simulink model "gm_parallel_8_prediction_and_cost_function"  (R2022a)
settings: Solver=FixedStepDiscrete  StartTime=0.0  StopTime=10.0  RelTol=1e-3
undefined symbols (not defined in the file or in its folder): f_c, L_d, L_q, L_x, L_y, p, psi_pm, R_ph
libraries: hdlmdlgenlib x42, hdlsllib x5
(part 1 of 7)
settings Model: Creator=Andre Merx  LastModifiedBy=Andre Merx
settings SolverCC: AlgebraicLoopSolver=TrustRegion
settings DataIOCC: LimitDataPoints=on  SaveOutput=off  SaveTime=off
settings OptimizationCC: BlockReduction=off  ConditionallyExecuteInputs=off  DefaultParameterBehavior=Inlined  LifeSpan=inf
settings DebuggingCC: AlgebraicLoopMsg=error  InheritedTsInSrcMsg=none  SingleTaskRateTransMsg=error  UnconnectedInputMsg=warning  UnconnectedOutputMsg=warning  UnconnectedLineMsg=warning  AllowSymbolicDim=off  StrictBusMsg=ErrorOnBusTreatedAsVector  SFUnexpectedBacktrackingDiag=warning  SFNoUnconditionalDefaultTransitionDiag=warning  SFExecutionAtInitializationDiag=none  SFMachineParentedDataDiag=warning  ArithmeticOperatorsInVariantConditions=warning
settings HardwareCC: ProdBitPerPointer=32  ProdBitPerSizeT=32  ProdBitPerPtrDiffT=32  ProdLargestAtomicFloat=None  ProdIntDivRoundTo=Undefined  ProdEndianess=Unspecified  ProdWordSize=32  ProdHWDeviceType=ASIC/FPGA->ASIC/FPGA  ProdEqTarget=off
settings SFSimCC: SimUseLocalCustomCode=off  CustomCodeUndefinedFunction=UseInterfaceOnly
settings RTWCC: RTWUseLocalCustomCode=off
settings CodeAppCC: StateflowObjectComments=on
settings GRTTargetCC: TargetLangStandard=C89/C90 (ANSI)
settings ConfigComp: CovScope=ReferencedModels  CovMetricSettings=dw  CovSaveCumulativeToWorkspaceVar=on  CovSaveSingleToWorkspaceVar=on  CovExternalEMLEnable=off  CovSFcnEnable=off

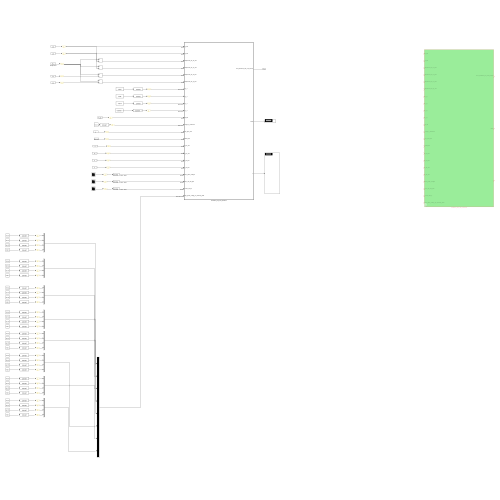
[thumbnail: Simulink's stored preview of the top-level diagram]
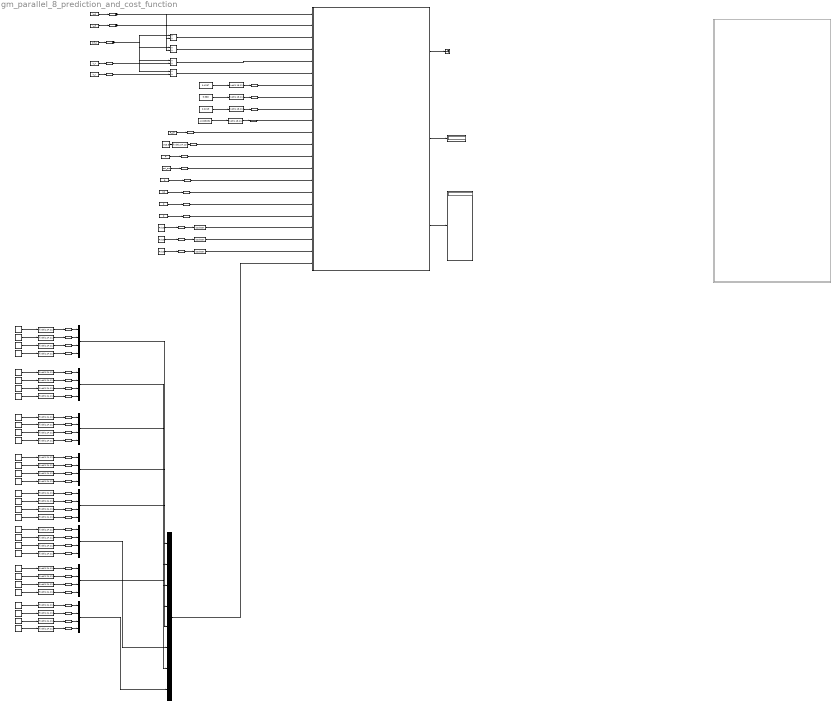
== system gm_parallel_8_prediction_and_cost_function ==
  Constant1 : Constant  Value=L_d  OutDataTypeStr=single  SampleTime=-1
  Constant10 : Constant  Value=0  OutDataTypeStr=single  SampleTime=-1
  Constant{11,30,34,38,42,46,70,74} (8 alike) : Constant  Value=-163.1
  Constant12 : Constant  Value=L_x  OutDataTypeStr=single  SampleTime=-1
  Constant13 : Constant  Value=L_y  OutDataTypeStr=single  SampleTime=-1
  Constant18 : Constant  Value=0.4297
  Constant19 : Constant  Value=R_ph  OutDataTypeStr=single  SampleTime=-1
  Constant2 : Constant  Value=L_q  OutDataTypeStr=single  SampleTime=-1
  Constant20 : Constant  Value=313.3
  Constant21 : Constant  Value=p  OutDataTypeStr=single  SampleTime=-1
  Constant22 : Constant  Value=9.988
  Constant23 : Constant  Value=0.2219
  Constant24 : Constant  Value=psi_pm  OutDataTypeStr=single  SampleTime=-1
  Constant25 : Constant  Value=-0.003051
  Constant{4,31,35,39,43,47,71,75} (8 alike) : Constant  Value=173.9
  Constant{5,32,36,40,44,48,72,76} (8 alike) : Constant  Value=72.19
  Constant{6,33,37,41,45,49,73,77} (8 alike) : Constant  Value=-94.17
  Constant7 : Constant  Value=0  OutDataTypeStr=single  SampleTime=-1
  Constant8 : Constant  Value=10  OutDataTypeStr=single  SampleTime=-1
  Constant9 : Constant  Value=0  OutDataTypeStr=single  SampleTime=-1
  Data Type Conversion{2..6,10,20..21,25..41,62..69} (33 alike) : DataTypeConversion  OutDataTypeStr=fixdt(1,24,11)  SaturateOnIntegerOverflow=off  RndMeth=Floor
  Data Type Conversion{12..15} (4 alike) : DataTypeConversion  OutDataTypeStr=fixdt(1,18,11)  SaturateOnIntegerOverflow=off  RndMeth=Floor
  Data Type Conversion22 : DataTypeConversion  OutDataTypeStr=boolean  SaturateOnIntegerOverflow=off  RndMeth=Floor
  Data Type Conversion23 : DataTypeConversion  OutDataTypeStr=boolean  SaturateOnIntegerOverflow=off  RndMeth=Floor
  Data Type Conversion24 : DataTypeConversion  OutDataTypeStr=boolean  SaturateOnIntegerOverflow=off  RndMeth=Floor
  Display : Display
  Display1 : Display
  Divide{,1..3} (4 alike) : Product  Inputs=*/  RndMeth=Zero  SaturateOnIntegerOverflow=on
  Mux{,1..7} (8 alike) : Mux
  Mux16 : Mux  Inputs=8
  Prediction_and_cost_function1 : Subsystem  TreatAsAtomicUnit=on
  Prediction_and_cost_function2 : Subsystem  Commented=on  TreatAsAtomicUnit=on
  Pulse Generator4 : DiscretePulseGenerator  PulseType=Time based  Period=1/f_c
  Pulse Generator5 : DiscretePulseGenerator  PulseType=Time based  Period=1/f_c
  Pulse Generator6 : DiscretePulseGenerator  PulseType=Time based  Period=1/f_c
  Rate Transition{3..8,12..15,17..28,33..54,75..82} (52 alike) : RateTransition  OutPortSampleTime=Rt
  SampleTime : Constant  Value=1/f_c  OutDataTypeStr=single  SampleTime=-1
  Terminator : Terminator
  wires:
  Mux5/1 -> Mux16/6
  Constant13/1 -> Rate Transition21/1
  SampleTime/1 -> Rate Transition19/1
  Rate Transition20/1 -> Divide2/2
  Constant49/1 -> Data Type Conversion40/1
  Data Type Conversion24/1 -> Prediction_and_cost_function1/19(done_phase_voltages)  "curent_valid_in"
  Constant4/1 -> Data Type Conversion10/1
  Constant18/1 -> Data Type Conversion12/1
  Divide/1 -> Prediction_and_cost_function1/3(SampleTime_div_Ld_AXI)
  Constant10/1 -> Rate Transition15/1
  Constant1/1 -> Rate Transition5/1
  Constant25/1 -> Data Type Conversion15/1
  Constant31/1 -> Data Type Conversion3/1
  Rate Transition33/1 -> Mux1/2
  Data Type Conversion10/1 -> Rate Transition3/1
  Divide3/1 -> Prediction_and_cost_function1/6(SampleTime_div_Ly_AXI)
  Rate Transition28/1 -> Prediction_and_cost_function1/10(iy_k_1)
  Rate Transition26/1 -> Prediction_and_cost_function1/9(ix_k_1)
  Constant6/1 -> Data Type Conversion4/1
  Constant8/1 -> Rate Transition13/1
  Data Type Conversion40/1 -> Rate Transition53/1
  Constant39/1 -> Data Type Conversion30/1
  Rate Transition27/1 -> Prediction_and_cost_function1/14(psiPM_AXI)
  Rate Transition21/1 -> Divide3/2
  Data Type Conversion15/1 -> Rate Transition28/1
  Constant7/1 -> Rate Transition12/1
  Rate Transition37/1 -> Data Type Conversion23/1
  Data Type Conversion22/1 -> Prediction_and_cost_function1/20(done_vsd_and_park)  "curent_valid_in"
  Rate Transition17/1 -> Prediction_and_cost_function1/7(id_k_1)
  Pulse Generator6/1 -> Rate Transition37/1
  Rate Transition36/1 -> Data Type Conversion22/1
  Constant47/1 -> Data Type Conversion38/1
  Rate Transition8/1 -> Mux/4
  Pulse Generator5/1 -> Rate Transition36/1
  Data Type Conversion34/1 -> Rate Transition47/1
  Rate Transition13/1 -> Prediction_and_cost_function1/16(iq_ref_AXI)
  Data Type Conversion14/1 -> Rate Transition26/1
  Constant77/1 -> Data Type Conversion68/1
  Rate Transition19/1 -> Divide/1, Divide2/1, Divide3/1, Divide1/1
  Pulse Generator4/1 -> Rate Transition35/1
  Constant22/1 -> Data Type Conversion13/1
  Data Type Conversion25/1 -> Rate Transition38/1
  Data Type Conversion31/1 -> Rate Transition44/1
  Constant20/1 -> Data Type Conversion5/1
  Data Type Conversion21/1 -> Rate Transition34/1
  Data Type Conversion20/1 -> Rate Transition33/1
  Rate Transition46/1 -> Mux4/4
  Constant35/1 -> Data Type Conversion26/1
  Data Type Conversion35/1 -> Rate Transition48/1
  Constant34/1 -> Data Type Conversion29/1
  Data Type Conversion33/1 -> Rate Transition46/1
  Data Type Conversion32/1 -> Rate Transition45/1
  Constant11/1 -> Data Type Conversion6/1
  Rate Transition3/1 -> Mux/1
  Constant36/1 -> Data Type Conversion27/1
  Data Type Conversion39/1 -> Rate Transition52/1
  Data Type Conversion27/1 -> Rate Transition40/1
  Rate Transition79/1 -> Mux6/1
  Data Type Conversion30/1 -> Rate Transition43/1
  Data Type Conversion37/1 -> Rate Transition50/1
  Data Type Conversion41/1 -> Rate Transition54/1
  Constant48/1 -> Data Type Conversion39/1
  Constant45/1 -> Data Type Conversion36/1
  Constant44/1 -> Data Type Conversion35/1
  Constant43/1 -> Data Type Conversion34/1
  Constant32/1 -> Data Type Conversion20/1
  Data Type Conversion12/1 -> Rate Transition17/1
  Rate Transition35/1 -> Data Type Conversion24/1
  Rate Transition41/1 -> Mux2/3
  Rate Transition78/1 -> Mux7/4
  Constant33/1 -> Data Type Conversion21/1
  Constant30/1 -> Data Type Conversion25/1
  Constant40/1 -> Data Type Conversion31/1
  Constant71/1 -> Data Type Conversion62/1
  Constant70/1 -> Data Type Conversion65/1
  Data Type Conversion4/1 -> Rate Transition7/1
  Data Type Conversion62/1 -> Rate Transition75/1
  Data Type Conversion67/1 -> Rate Transition80/1
  Data Type Conversion69/1 -> Rate Transition82/1
  Data Type Conversion13/1 -> Rate Transition25/1
  Constant2/1 -> Rate Transition6/1
  Rate Transition14/1 -> Prediction_and_cost_function1/17(ix_ref_AXI)
  Data Type Conversion63/1 -> Rate Transition76/1
  Constant21/1 -> Rate Transition24/1
  Constant76/1 -> Data Type Conversion67/1
  Rate Transition25/1 -> Prediction_and_cost_function1/8(iq_k_1)
  Constant74/1 -> Data Type Conversion69/1
  Constant75/1 -> Data Type Conversion66/1
  Data Type Conversion68/1 -> Rate Transition81/1
  Rate Transition18/1 -> Mux1/1
  Constant38/1 -> Data Type Conversion33/1
  Rate Transition7/1 -> Mux/3
  Constant41/1 -> Data Type Conversion32/1
  Data Type Conversion6/1 -> Rate Transition8/1
  Rate Transition23/1 -> Prediction_and_cost_function1/12(omega_m_measured)
  Data Type Conversion66/1 -> Rate Transition79/1
  Constant37/1 -> Data Type Conversion28/1
  Constant23/1 -> Data Type Conversion14/1
  Constant12/1 -> Rate Transition20/1
  Rate Transition15/1 -> Prediction_and_cost_function1/18(iy_ref_AXI)
  Constant73/1 -> Data Type Conversion64/1
  Constant19/1 -> Rate Transition22/1
  Data Type Conversion28/1 -> Rate Transition41/1
  Constant9/1 -> Rate Transition14/1
  Rate Transition39/1 -> Mux2/1
  Rate Transition40/1 -> Mux2/2
  Constant46/1 -> Data Type Conversion41/1
  Rate Transition82/1 -> Mux6/4
  Mux7/1 -> Mux16/8
  Rate Transition5/1 -> Divide/2, Prediction_and_cost_function1/2(Ld_AXI)
  Data Type Conversion23/1 -> Prediction_and_cost_function1/21(current_valid_in)  "curent_valid_in"
  Prediction_and_cost_function1/1(done_Prediction_and_cost_function) -> Terminator/1
  Mux4/1 -> Mux16/5
  Rate Transition42/1 -> Mux2/4
  Prediction_and_cost_function1/2(Index) -> Display/1
  Rate Transition47/1 -> Mux3/1
  Data Type Conversion36/1 -> Rate Transition49/1
  Rate Transition49/1 -> Mux3/3
  Rate Transition43/1 -> Mux4/1
  Rate Transition12/1 -> Prediction_and_cost_function1/15(id_ref_AXI)
  Rate Transition80/1 -> Mux6/2
  Rate Transition6/1 -> Divide1/2, Prediction_and_cost_function1/1(Lq_AXI)
  Rate Transition52/1 -> Mux5/2
  Constant24/1 -> Rate Transition27/1
  Data Type Conversion38/1 -> Rate Transition51/1
  Rate Transition50/1 -> Mux3/4
  Constant42/1 -> Data Type Conversion37/1
  Rate Transition76/1 -> Mux7/2
  Data Type Conversion3/1 -> Rate Transition18/1
  Constant5/1 -> Data Type Conversion2/1
  Data Type Conversion26/1 -> Rate Transition39/1
  Rate Transition45/1 -> Mux4/3
  Rate Transition53/1 -> Mux5/3
  Rate Transition54/1 -> Mux5/4
  Rate Transition77/1 -> Mux7/3
  Rate Transition4/1 -> Mux/2
  Data Type Conversion64/1 -> Rate Transition77/1
  Divide1/1 -> Prediction_and_cost_function1/4(SampleTime_div_Lq_AXI)
  Rate Transition75/1 -> Mux7/1
  Mux3/1 -> Mux16/4
  Rate Transition44/1 -> Mux4/2
  Data Type Conversion65/1 -> Rate Transition78/1
  Mux/1 -> Mux16/1
  Rate Transition38/1 -> Mux1/4
  Rate Transition48/1 -> Mux3/2
  Rate Transition81/1 -> Mux6/3
  Data Type Conversion2/1 -> Rate Transition4/1
  Divide2/1 -> Prediction_and_cost_function1/5(SampleTime_div_Lx_AXI)
  Mux1/1 -> Mux16/2
  Constant72/1 -> Data Type Conversion63/1
  Rate Transition22/1 -> Prediction_and_cost_function1/11(Rs_AXI)
  Mux6/1 -> Mux16/7
  Mux16/1 -> Prediction_and_cost_function1/22(dqxy_phase_voltage_per_switching_state)
  Rate Transition34/1 -> Mux1/3
  Rate Transition51/1 -> Mux5/1
  Rate Transition24/1 -> Prediction_and_cost_function1/13(pole_pairs_AXI)
  Data Type Conversion29/1 -> Rate Transition42/1
  Data Type Conversion5/1 -> Rate Transition23/1
  Prediction_and_cost_function1/3(J) -> Display1/1
  Mux2/1 -> Mux16/3

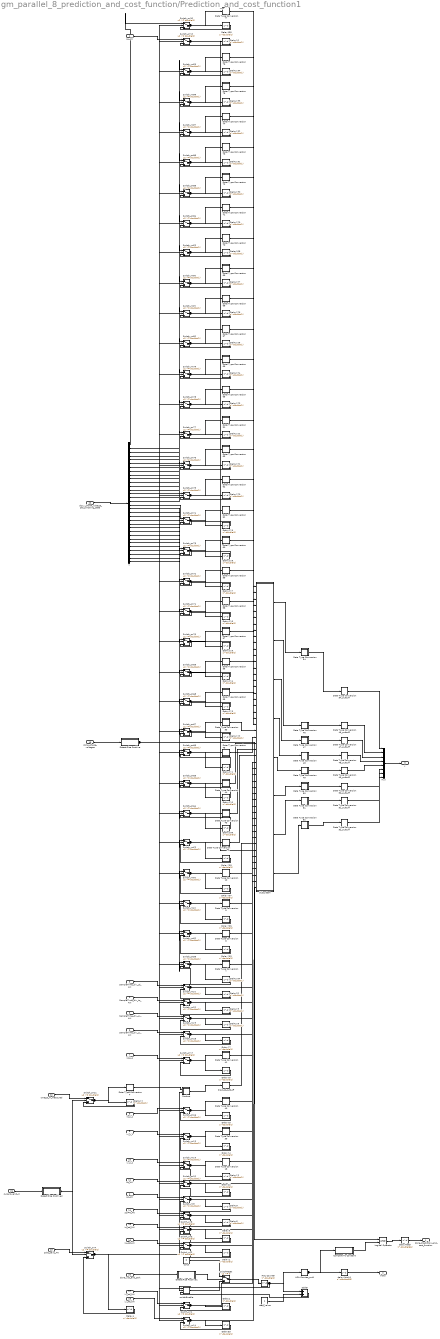
== system gm_parallel_8_prediction_and_cost_function/Prediction_and_cost_function1 ==
  Lq_AXI : Inport  OutDataTypeStr=single  PortDimensions=1  SampleTime=1e-08
  Ld_AXI : Inport  Port=2  OutDataTypeStr=single  PortDimensions=1  SampleTime=1e-08
  SampleTime_div_Ld_AXI : Inport  Port=3  OutDataTypeStr=single  PortDimensions=1  SampleTime=1e-08
  SampleTime_div_Lq_AXI : Inport  Port=4  OutDataTypeStr=single  PortDimensions=1  SampleTime=1e-08
  SampleTime_div_Lx_AXI : Inport  Port=5  OutDataTypeStr=single  PortDimensions=1  SampleTime=1e-08
  SampleTime_div_Ly_AXI : Inport  Port=6  OutDataTypeStr=single  PortDimensions=1  SampleTime=1e-08
  id_k_1 : Inport  Port=7  OutDataTypeStr=fixdt(1, 18, 11)  PortDimensions=1  SampleTime=1e-08
  iq_k_1 : Inport  Port=8  OutDataTypeStr=fixdt(1, 18, 11)  PortDimensions=1  SampleTime=1e-08
  ix_k_1 : Inport  Port=9  OutDataTypeStr=fixdt(1, 18, 11)  PortDimensions=1  SampleTime=1e-08
  iy_k_1 : Inport  Port=10  OutDataTypeStr=fixdt(1, 18, 11)  PortDimensions=1  SampleTime=1e-08
  Rs_AXI : Inport  Port=11  OutDataTypeStr=single  PortDimensions=1  SampleTime=1e-08
  omega_m_measured : Inport  Port=12  OutDataTypeStr=fixdt(1, 24, 11)  PortDimensions=1  SampleTime=1e-08
  pole_pairs_AXI : Inport  Port=13  OutDataTypeStr=single  PortDimensions=1  SampleTime=1e-08
  psiPM_AXI : Inport  Port=14  OutDataTypeStr=single  PortDimensions=1  SampleTime=1e-08
  id_ref_AXI : Inport  Port=15  OutDataTypeStr=single  PortDimensions=1  SampleTime=1e-08
  iq_ref_AXI : Inport  Port=16  OutDataTypeStr=single  PortDimensions=1  SampleTime=1e-08
  ix_ref_AXI : Inport  Port=17  OutDataTypeStr=single  PortDimensions=1  SampleTime=1e-08
  iy_ref_AXI : Inport  Port=18  OutDataTypeStr=single  PortDimensions=1  SampleTime=1e-08
  done_phase_voltages : Inport  Port=19  OutDataTypeStr=boolean  PortDimensions=1  SampleTime=1e-08
  done_vsd_and_park : Inport  Port=20  OutDataTypeStr=boolean  PortDimensions=1  SampleTime=1e-08
  current_valid_in : Inport  Port=21  OutDataTypeStr=boolean  PortDimensions=1  SampleTime=1e-08
  dqxy_phase_voltage_per_switching_state : Inport  Port=22  OutDataTypeStr=fixdt(1, 24, 11)  PortDimensions=[32]  SampleTime=1e-08
  Compare To Constant : Subsystem  mask(Compare To Constant){relop=<=, const=double(8), OutDataTypeStr=boolean, ZeroCross=on}
      mask prompts: relop "Simulink:masks:Operator_MP"; const "Simulink:masks:ConstantValue_MP"; OutDataTypeStr "Simulink:masks:OutputDataType_MP"; ZeroCross "Simulink:masks:EnableZerocrossingDetection_MP"
      mask help: Simulink:masks:CompareToConstant_MD
      mask init:
      | OutDataTypeStr = 'boolean';
      | ZeroCross = 'on';
      | blkName = 'parallel_8_prediction_and_cost_function/Prediction_and_cost_function1/Compare\nTo Constant';
      | const = double(8);
      | const_str = '8';
      | const_val = double(8);
      | relop = '<=';
      | setValue = 'boolean';
      | str = '<= 8';
      mask TypeOptions relop: == | ~= | < | <= | >= | >
      mask TypeOptions OutDataTypeStr: Simulink:masks:uint8 | Simulink:masks:boolean
      mask Callback ZeroCross: sl('zeroCrossEnable', gcbh);
      mask Display: disp(str)
  Data Type Conversion10 : Subsystem
      mask Display: disp('NFP\nconv');
  Data Type Conversion18 : Subsystem
      mask Display: disp('NFP\nconv');
  Data Type Conversion39 : Subsystem
      mask Display: disp('NFP\nconv');
  Data Type Conversion4 : Subsystem
      mask Display: disp('NFP\nconv');
  Data Type Conversion40 : Subsystem
      mask Display: disp('NFP\nconv');
  Data Type Conversion41 : Subsystem
      mask Display: disp('NFP\nconv');
  Data Type Conversion42 : Subsystem
      mask Display: disp('NFP\nconv');
  Data Type Conversion43 : Subsystem
      mask Display: disp('NFP\nconv');
  Data Type Conversion44 : Subsystem
      mask Display: disp('NFP\nconv');
  Data Type Conversion45 : Subsystem
      mask Display: disp('NFP\nconv');
  Data Type Conversion46 : Subsystem
      mask Display: disp('NFP\nconv');
  Data Type Conversion46_outbuff : hdlmdlgenlib/Buffer
      settings: SourceProductBaseCode=SL
  Data Type Conversion47 : Subsystem
      mask Display: disp('NFP\nconv');
  Data Type Conversion47_outbuff : hdlmdlgenlib/Buffer
      settings: SourceProductBaseCode=SL
  Data Type Conversion48 : Subsystem
      mask Display: disp('NFP\nconv');
  Data Type Conversion48_outbuff : hdlmdlgenlib/Buffer
      settings: SourceProductBaseCode=SL
  Data Type Conversion49 : Subsystem
      mask Display: disp('NFP\nconv');
  Data Type Conversion49_outbuff : hdlmdlgenlib/Buffer
      settings: SourceProductBaseCode=SL
  Data Type Conversion50 : Subsystem
      mask Display: disp('NFP\nconv');
  Data Type Conversion50_outbuff : hdlmdlgenlib/Buffer
      settings: SourceProductBaseCode=SL
  Data Type Conversion51 : Subsystem
      mask Display: disp('NFP\nconv');
  Data Type Conversion51_outbuff : hdlmdlgenlib/Buffer
      settings: SourceProductBaseCode=SL
  Data Type Conversion52 : Subsystem
      mask Display: disp('NFP\nconv');
  Data Type Conversion52_outbuff : hdlmdlgenlib/Buffer
      settings: SourceProductBaseCode=SL
  Data Type Conversion53 : Subsystem
      mask Display: disp('NFP\nconv');
  Data Type Conversion54 : Subsystem
      mask Display: disp('NFP\nconv');
  Data Type Conversion54_outbuff : hdlmdlgenlib/Buffer
      settings: SourceProductBaseCode=SL
  Data Type Conversion55 : Subsystem
      mask Display: disp('NFP\nconv');
  Data Type Conversion56 : Subsystem
      mask Display: disp('NFP\nconv');
  Data Type Conversion57 : Subsystem
      mask Display: disp('NFP\nconv');
  Data Type Conversion58 : Subsystem
      mask Display: disp('NFP\nconv');
  Data Type Conversion59 : Subsystem
      mask Display: disp('NFP\nconv');
  Data Type Conversion60 : Subsystem
      mask Display: disp('NFP\nconv');
  Data Type Conversion61 : Subsystem
      mask Display: disp('NFP\nconv');
  Data Type Conversion62 : Subsystem
      mask Display: disp('NFP\nconv');
  Data Type Conversion63 : Subsystem
      mask Display: disp('NFP\nconv');
  Data Type Conversion64 : Subsystem
      mask Display: disp('NFP\nconv');
  Data Type Conversion65 : Subsystem
      mask Display: disp('NFP\nconv');
  Data Type Conversion66 : Subsystem
      mask Display: disp('NFP\nconv');
  Data Type Conversion67 : Subsystem
      mask Display: disp('NFP\nconv');
  Data Type Conversion68 : Subsystem
      mask Display: disp('NFP\nconv');
  Data Type Conversion69 : Subsystem
      mask Display: disp('NFP\nconv');
  Data Type Conversion7 : Subsystem
      mask Display: disp('NFP\nconv');
  Data Type Conversion70 : Subsystem
      mask Display: disp('NFP\nconv');
  Data Type Conversion71 : Subsystem
      mask Display: disp('NFP\nconv');
  Data Type Conversion72 : Subsystem
      mask Display: disp('NFP\nconv');
  Data Type Conversion73 : Subsystem
      mask Display: disp('NFP\nconv');
  Data Type Conversion74 : Subsystem
      mask Display: disp('NFP\nconv');
  Data Type Conversion75 : Subsystem
      mask Display: disp('NFP\nconv');
  Data Type Conversion76 : Subsystem
      mask Display: disp('NFP\nconv');
  Data Type Conversion77 : Subsystem
      mask Display: disp('NFP\nconv');
  Data Type Conversion8 : Subsystem
      mask Display: disp('NFP\nconv');
  Data Type Conversion9 : Subsystem
      mask Display: disp('NFP\nconv');
  Delay{1..4,8..20,33,104..135} (50 alike) : Delay  DelayLength=double(1)  InitialCondition=0  SampleTime=1e-08
  Detect Rise Positive : Subsystem  mask(Detect Rise Positive){vinit=double(0), InputProcessing=Elements as channels (sample based), OutDataTypeStr=boolean}
      mask prompts: vinit "Simulink:masks:InitialCondition_MP"; InputProcessing "Simulink:masks:InputProcessing_MP"; OutDataTypeStr "Simulink:masks:OutputDataType_MP"
      mask help: Simulink:masks:DetectRisePositive_MD
      mask init:
      | InputProcessing = 'Elements as channels (sample based)';
      | OutDataTypeStr = 'boolean';
      | vinit = double(0);
      mask TypeOptions InputProcessing: Simulink:masks:ColumnsAsChannelsFrameBased | Simulink:masks:ElementsAsChannelsSampleBased
      mask TypeOptions OutDataTypeStr: Simulink:masks:uint8 | Simulink:masks:boolean
      mask Display: fprintf('U > 0\n&  NOT\nU/z > 0')
  Detect Rise Positive1 : Subsystem  mask(Detect Rise Positive){vinit=double(0), InputProcessing=Elements as channels (sample based), OutDataTypeStr=boolean}
      mask prompts: vinit "Simulink:masks:InitialCondition_MP"; InputProcessing "Simulink:masks:InputProcessing_MP"; OutDataTypeStr "Simulink:masks:OutputDataType_MP"
      mask help: Simulink:masks:DetectRisePositive_MD
      mask init:
      | InputProcessing = 'Elements as channels (sample based)';
      | OutDataTypeStr = 'boolean';
      | vinit = double(0);
      mask TypeOptions InputProcessing: Simulink:masks:ColumnsAsChannelsFrameBased | Simulink:masks:ElementsAsChannelsSampleBased
      mask TypeOptions OutDataTypeStr: Simulink:masks:uint8 | Simulink:masks:boolean
      mask Display: fprintf('U > 0\n&  NOT\nU/z > 0')
  Detect Rise Positive2 : Subsystem  mask(Detect Rise Positive){vinit=double(0), InputProcessing=Elements as channels (sample based), OutDataTypeStr=boolean}
      mask prompts: vinit "Simulink:masks:InitialCondition_MP"; InputProcessing "Simulink:masks:InputProcessing_MP"; OutDataTypeStr "Simulink:masks:OutputDataType_MP"
      mask help: Simulink:masks:DetectRisePositive_MD
      mask init:
      | InputProcessing = 'Elements as channels (sample based)';
      | OutDataTypeStr = 'boolean';
      | vinit = double(0);
      mask TypeOptions InputProcessing: Simulink:masks:ColumnsAsChannelsFrameBased | Simulink:masks:ElementsAsChannelsSampleBased
      mask TypeOptions OutDataTypeStr: Simulink:masks:uint8 | Simulink:masks:boolean
      mask Display: fprintf('U > 0\n&  NOT\nU/z > 0')
  HDL Counter : Delay  DelayLength=double(1)  InitialCondition=0  SampleTime=1e-08
  HDL Counter_out1 : hdlmdlgenlib/Buffer
      settings: SourceProductBaseCode=SL
  Logical Operator : Logic  AllPortsSameDT=off  OutDataTypeStr=boolean  SampleTime=1e-08
  Product : Subsystem
      mask Display: disp('NFP\nmul');
  Product_outbuff : hdlmdlgenlib/Buffer
      settings: SourceProductBaseCode=SL
  Subsystem : Subsystem
  Switch_on{1..4,8..10,12,14,18..21} (13 alike) : Switch  Threshold=double(1)  OutDataTypeStr=single  RndMeth=Simplest  SampleTime=1e-08  SaturateOnIntegerOverflow=off  InputSameDT=off
  Switch_on{11,59..90} (33 alike) : Switch  Threshold=double(1)  OutDataTypeStr=fixdt(1, 24, 11)  RndMeth=Simplest  SampleTime=1e-08  SaturateOnIntegerOverflow=off  InputSameDT=off
  Switch_on{13,15..17} (4 alike) : Switch  Threshold=double(1)  OutDataTypeStr=fixdt(1, 18, 11)  RndMeth=Simplest  SampleTime=1e-08  SaturateOnIntegerOverflow=off  InputSameDT=off
  adder : Sum  AccumDataTypeStr=int32  OutDataTypeStr=int32  SampleTime=1e-08
  const : Constant  Value=0  VectorParams1D=off  OutDataTypeStr=int32  SampleTime=1e-08
  delayMatch : Delay  DelayLength=double(66)  InitialCondition=0  SampleTime=1e-08
  delayMatch1 : Delay  DelayLength=double(66)  InitialCondition=0  SampleTime=1e-08
  mux : Mux  Inputs=8
  step_value : Constant  VectorParams1D=off  OutDataTypeStr=int32  SampleTime=1e-08
  switchEnable : MultiPortSwitch  DataPortOrder=Zero-based contiguous  Inputs=2  DiagnosticForDefault=None  zeroidx=on  OutDataTypeStr=int32  SampleTime=1e-08  SaturateOnIntegerOverflow=off  InputSameDT=off
  switchReset : Switch  Criteria=u2 ~= 0  Threshold=double(0)  OutDataTypeStr=int32  SampleTime=1e-08  SaturateOnIntegerOverflow=off  InputSameDT=off
  t : Demux  Outputs=32
  done_Prediction_and_cost_function : Outport  SampleTime=1e-08
  Index : Outport  Port=2  SampleTime=1e-08
  J : Outport  Port=3  SampleTime=1e-08
  wires:
  Lq_AXI/1 -> Switch_on10/1
  Ld_AXI/1 -> Switch_on9/1
  SampleTime_div_Ld_AXI/1 -> Switch_on21/1
  SampleTime_div_Lq_AXI/1 -> Switch_on20/1
  SampleTime_div_Lx_AXI/1 -> Switch_on19/1
  SampleTime_div_Ly_AXI/1 -> Switch_on18/1
  id_k_1/1 -> Switch_on17/1
  iq_k_1/1 -> Switch_on16/1
  ix_k_1/1 -> Switch_on15/1
  iy_k_1/1 -> Switch_on13/1
  Rs_AXI/1 -> Switch_on12/1
  omega_m_measured/1 -> Switch_on11/1
  pole_pairs_AXI/1 -> Switch_on4/1
  psiPM_AXI/1 -> Switch_on8/1
  id_ref_AXI/1 -> Switch_on3/1
  iq_ref_AXI/1 -> Switch_on2/1
  ix_ref_AXI/1 -> Switch_on1/1
  iy_ref_AXI/1 -> Switch_on14/1
  done_phase_voltages/1 -> Detect Rise Positive/1(U)
  done_vsd_and_park/1 -> Detect Rise Positive1/1(U)
  current_valid_in/1 -> Detect Rise Positive2/1(U)
  dqxy_phase_voltage_per_switching_state/1 -> t/1
  Compare To Constant/1(y) -> Logical Operator/2
  Data Type Conversion46_outbuff/1 -> mux/2
  Data Type Conversion47_outbuff/1 -> mux/3
  Data Type Conversion48_outbuff/1 -> mux/4
  Data Type Conversion49_outbuff/1 -> mux/5
  Data Type Conversion50_outbuff/1 -> mux/6
  Data Type Conversion51_outbuff/1 -> mux/7
  Data Type Conversion52_outbuff/1 -> mux/8
  Data Type Conversion54_outbuff/1 -> mux/1
  Detect Rise Positive/1(Y) -> Logical Operator/1, switchEnable/1, Switch_on90/2, Switch_on89/2, Switch_on88/2, Switch_on87/2, Switch_on86/2, Switch_on85/2, Switch_on84/2, Switch_on83/2, Switch_on82/2, Switch_on81/2, Switch_on80/2, Switch_on79/2, Switch_on78/2, Switch_on77/2, Switch_on76/2, Switch_on75/2, Switch_on74/2, Switch_on73/2, Switch_on72/2, Switch_on71/2, Switch_on70/2, Switch_on69/2, Switch_on68/2, Switch_on67/2, Switch_on66/2, Switch_on65/2, Switch_on64/2, Switch_on63/2, Switch_on62/2, Switch_on61/2, Switch_on60/2, Switch_on59/2, Switch_on21/2, Switch_on20/2, Switch_on19/2, Switch_on18/2, Switch_on17/2, Switch_on16/2, Switch_on15/2, Switch_on13/2, Switch_on12/2, Switch_on10/2, Switch_on9/2, Switch_on8/2, Switch_on3/2, Switch_on2/2, Switch_on1/2, Switch_on14/2
  Detect Rise Positive1/1(Y) -> switchReset/2
  Detect Rise Positive2/1(Y) -> Switch_on11/2, Switch_on4/2
  delayMatch1/1 -> Index/1
  delayMatch/1 -> done_Prediction_and_cost_function/1
  mux/1 -> J/1
  Product_outbuff/1 -> Subsystem/42(omega_el15)
  Subsystem/1(J) -> Data Type Conversion54/1(In1)
  Subsystem/2(J1) -> Data Type Conversion46/1(In1)
  Subsystem/3(J2) -> Data Type Conversion47/1(In1)
  Subsystem/4(J3) -> Data Type Conversion48/1(In1)
  Subsystem/5(J4) -> Data Type Conversion49/1(In1)
  Subsystem/6(J5) -> Data Type Conversion50/1(In1)
  Subsystem/7(J6) -> Data Type Conversion51/1(In1)
  Subsystem/8(J7) -> Data Type Conversion52/1(In1)
  Switch_on1/1 -> Subsystem/48(ix_ref15), Delay1/1
  Switch_on10/1 -> Subsystem/43(Lq15), Delay10/1
  Switch_on11/1 -> Data Type Conversion4/1(In1), Delay11/1
  Switch_on12/1 -> Subsystem/41(Rs15), Delay12/1
  Switch_on13/1 -> Data Type Conversion18/1(In1), Delay13/1
  Switch_on14/1 -> Subsystem/49(iy_ref15), Delay33/1
  Switch_on15/1 -> Data Type Conversion39/1(In1), Delay14/1
  Switch_on16/1 -> Data Type Conversion40/1(In1), Delay15/1
  Switch_on17/1 -> Data Type Conversion41/1(In1), Delay16/1
  Switch_on18/1 -> Subsystem/36(SampleTime_div_Ly15), Delay17/1
  Switch_on19/1 -> Subsystem/35(SampleTime_div_Lx15), Delay18/1
  Switch_on2/1 -> Subsystem/47(iq_ref15), Delay2/1
  Switch_on20/1 -> Subsystem/34(SampleTime_div_Lq15), Delay19/1
  Switch_on21/1 -> Subsystem/33(SampleTime_div_Ld15), Delay20/1
  Switch_on3/1 -> Subsystem/46(id_ref15), Delay3/1
  Switch_on4/1 -> Product/2(In2), Delay4/1
  Switch_on59/1 -> Data Type Conversion7/1(In1), Delay104/1
  Switch_on60/1 -> Data Type Conversion8/1(In1), Delay105/1
  Switch_on61/1 -> Data Type Conversion9/1(In1), Delay106/1
  Switch_on62/1 -> Data Type Conversion10/1(In1), Delay107/1
  Switch_on63/1 -> Data Type Conversion42/1(In1), Delay108/1
  Switch_on64/1 -> Data Type Conversion43/1(In1), Delay109/1
  Switch_on65/1 -> Data Type Conversion44/1(In1), Delay110/1
  Switch_on66/1 -> Data Type Conversion45/1(In1), Delay111/1
  Switch_on67/1 -> Data Type Conversion53/1(In1), Delay112/1
  Switch_on68/1 -> Data Type Conversion55/1(In1), Delay113/1
  Switch_on69/1 -> Data Type Conversion56/1(In1), Delay114/1
  Switch_on70/1 -> Data Type Conversion57/1(In1), Delay115/1
  Switch_on71/1 -> Data Type Conversion58/1(In1), Delay116/1
  Switch_on72/1 -> Data Type Conversion59/1(In1), Delay117/1
  Switch_on73/1 -> Data Type Conversion60/1(In1), Delay118/1
  Switch_on74/1 -> Data Type Conversion61/1(In1), Delay119/1
  Switch_on75/1 -> Data Type Conversion62/1(In1), Delay120/1
  Switch_on76/1 -> Data Type Conversion63/1(In1), Delay121/1
  Switch_on77/1 -> Data Type Conversion64/1(In1), Delay122/1
  Switch_on78/1 -> Data Type Conversion65/1(In1), Delay123/1
  Switch_on79/1 -> Data Type Conversion66/1(In1), Delay124/1
  Switch_on8/1 -> Subsystem/45(psiPM15), Delay8/1
  Switch_on80/1 -> Data Type Conversion67/1(In1), Delay125/1
  Switch_on81/1 -> Data Type Conversion68/1(In1), Delay126/1
  Switch_on82/1 -> Data Type Conversion69/1(In1), Delay127/1
  Switch_on83/1 -> Data Type Conversion70/1(In1), Delay128/1
  Switch_on84/1 -> Data Type Conversion71/1(In1), Delay129/1
  Switch_on85/1 -> Data Type Conversion72/1(In1), Delay130/1
  Switch_on86/1 -> Data Type Conversion73/1(In1), Delay131/1
  Switch_on87/1 -> Data Type Conversion74/1(In1), Delay132/1
  Switch_on88/1 -> Data Type Conversion75/1(In1), Delay133/1
  Switch_on89/1 -> Data Type Conversion76/1(In1), Delay134/1
  Switch_on9/1 -> Subsystem/44(Ld15), Delay9/1
  Switch_on90/1 -> Data Type Conversion77/1(In1), Delay135/1
  HDL Counter/1 -> HDL Counter_out1/1, switchEnable/2, adder/1
  const/1 -> switchReset/1
  step_value/1 -> adder/2
  t/1 -> Switch_on90/1
  t/2 -> Switch_on89/1
  t/3 -> Switch_on88/1
  t/4 -> Switch_on87/1
  t/5 -> Switch_on86/1
  t/6 -> Switch_on85/1
  t/7 -> Switch_on84/1
  t/8 -> Switch_on83/1
  t/9 -> Switch_on82/1
  t/10 -> Switch_on81/1
  t/11 -> Switch_on80/1
  t/12 -> Switch_on79/1
  t/13 -> Switch_on78/1
  t/14 -> Switch_on77/1
  t/15 -> Switch_on76/1
  t/16 -> Switch_on75/1
  t/17 -> Switch_on74/1
  t/18 -> Switch_on73/1
  t/19 -> Switch_on72/1
  t/20 -> Switch_on71/1
  t/21 -> Switch_on70/1
  t/22 -> Switch_on69/1
  t/23 -> Switch_on68/1
  t/24 -> Switch_on67/1
  t/25 -> Switch_on66/1
  t/26 -> Switch_on65/1
  t/27 -> Switch_on64/1
  t/28 -> Switch_on63/1
  t/29 -> Switch_on62/1
  t/30 -> Switch_on61/1
  t/31 -> Switch_on60/1
  t/32 -> Switch_on59/1
  Logical Operator/1 -> delayMatch/1
  HDL Counter_out1/1 -> delayMatch1/1, Compare To Constant/1(u)
  Data Type Conversion10/1(Out1) -> Subsystem/29(d_phase_voltage_per_switching_state7)
  Data Type Conversion18/1(Out1) -> Subsystem/40(iy_k_16)
  Data Type Conversion39/1(Out1) -> Subsystem/39(ix_k_16)
  Data Type Conversion4/1(Out1) -> Product/1(In1)
  Data Type Conversion40/1(Out1) -> Subsystem/38(iq_k_16)
  Data Type Conversion41/1(Out1) -> Subsystem/37(id_k_16)
  Data Type Conversion42/1(Out1) -> Subsystem/28(y_phase_voltage_per_switching_state6)
  Data Type Conversion43/1(Out1) -> Subsystem/27(x_phase_voltage_per_switching_state6)
  Data Type Conversion44/1(Out1) -> Subsystem/26(q_phase_voltage_per_switching_state6)
  Data Type Conversion45/1(Out1) -> Subsystem/25(d_phase_voltage_per_switching_state6)
  Data Type Conversion46/1(Out1) -> Data Type Conversion46_outbuff/1
  Data Type Conversion47/1(Out1) -> Data Type Conversion47_outbuff/1
  Data Type Conversion48/1(Out1) -> Data Type Conversion48_outbuff/1
  Data Type Conversion49/1(Out1) -> Data Type Conversion49_outbuff/1
  Data Type Conversion50/1(Out1) -> Data Type Conversion50_outbuff/1
  Data Type Conversion51/1(Out1) -> Data Type Conversion51_outbuff/1
  Data Type Conversion52/1(Out1) -> Data Type Conversion52_outbuff/1
  Data Type Conversion53/1(Out1) -> Subsystem/24(y_phase_voltage_per_switching_state5)
  Data Type Conversion54/1(Out1) -> Data Type Conversion54_outbuff/1
  Data Type Conversion55/1(Out1) -> Subsystem/23(x_phase_voltage_per_switching_state5)
  Data Type Conversion56/1(Out1) -> Subsystem/22(q_phase_voltage_per_switching_state5)
  Data Type Conversion57/1(Out1) -> Subsystem/21(d_phase_voltage_per_switching_state5)
  Data Type Conversion58/1(Out1) -> Subsystem/20(y_phase_voltage_per_switching_state4)
  Data Type Conversion59/1(Out1) -> Subsystem/19(x_phase_voltage_per_switching_state4)
  Data Type Conversion60/1(Out1) -> Subsystem/18(q_phase_voltage_per_switching_state4)
  Data Type Conversion61/1(Out1) -> Subsystem/17(d_phase_voltage_per_switching_state4)
  Data Type Conversion62/1(Out1) -> Subsystem/16(y_phase_voltage_per_switching_state3)
  Data Type Conversion63/1(Out1) -> Subsystem/15(x_phase_voltage_per_switching_state3)
  Data Type Conversion64/1(Out1) -> Subsystem/14(q_phase_voltage_per_switching_state3)
  Data Type Conversion65/1(Out1) -> Subsystem/13(d_phase_voltage_per_switching_state3)
  Data Type Conversion66/1(Out1) -> Subsystem/12(y_phase_voltage_per_switching_state2)
  Data Type Conversion67/1(Out1) -> Subsystem/11(x_phase_voltage_per_switching_state2)
  Data Type Conversion68/1(Out1) -> Subsystem/10(q_phase_voltage_per_switching_state2)
  Data Type Conversion69/1(Out1) -> Subsystem/9(d_phase_voltage_per_switching_state2)
  Data Type Conversion7/1(Out1) -> Subsystem/32(y_phase_voltage_per_switching_state7)
  Data Type Conversion70/1(Out1) -> Subsystem/8(y_phase_voltage_per_switching_state1)
  Data Type Conversion71/1(Out1) -> Subsystem/7(x_phase_voltage_per_switching_state1)
  Data Type Conversion72/1(Out1) -> Subsystem/6(q_phase_voltage_per_switching_state1)
  Data Type Conversion73/1(Out1) -> Subsystem/5(d_phase_voltage_per_switching_state1)
  Data Type Conversion74/1(Out1) -> Subsystem/4(y_phase_voltage_per_switching_state)
  Data Type Conversion75/1(Out1) -> Subsystem/3(x_phase_voltage_per_switching_state)
  Data Type Conversion76/1(Out1) -> Subsystem/2(q_phase_voltage_per_switching_state)
  Data Type Conversion77/1(Out1) -> Subsystem/1(d_phase_voltage_per_switching_state)
  Data Type Conversion8/1(Out1) -> Subsystem/31(x_phase_voltage_per_switching_state7)
  Data Type Conversion9/1(Out1) -> Subsystem/30(q_phase_voltage_per_switching_state7)
  Product/1(Out1) -> Product_outbuff/1
  adder/1 -> switchEnable/3
  switchEnable/1 -> switchReset/3
  switchReset/1 -> HDL Counter/1
  Delay135/1 -> Switch_on90/3
  Delay134/1 -> Switch_on89/3
  Delay133/1 -> Switch_on88/3
  Delay132/1 -> Switch_on87/3
  Delay131/1 -> Switch_on86/3
  Delay130/1 -> Switch_on85/3
  Delay129/1 -> Switch_on84/3
  Delay128/1 -> Switch_on83/3
  Delay127/1 -> Switch_on82/3
  Delay126/1 -> Switch_on81/3
  Delay125/1 -> Switch_on80/3
  Delay124/1 -> Switch_on79/3
  Delay123/1 -> Switch_on78/3
  Delay122/1 -> Switch_on77/3
  Delay121/1 -> Switch_on76/3
  Delay120/1 -> Switch_on75/3
  Delay119/1 -> Switch_on74/3
  Delay118/1 -> Switch_on73/3
  Delay117/1 -> Switch_on72/3
  Delay116/1 -> Switch_on71/3
  Delay115/1 -> Switch_on70/3
  Delay114/1 -> Switch_on69/3
  Delay113/1 -> Switch_on68/3
  Delay112/1 -> Switch_on67/3
  Delay111/1 -> Switch_on66/3
  Delay110/1 -> Switch_on65/3
  Delay109/1 -> Switch_on64/3
  Delay108/1 -> Switch_on63/3
  Delay107/1 -> Switch_on62/3
  Delay106/1 -> Switch_on61/3
  Delay105/1 -> Switch_on60/3
  Delay104/1 -> Switch_on59/3
  Delay20/1 -> Switch_on21/3
  Delay19/1 -> Switch_on20/3
  Delay18/1 -> Switch_on19/3
  Delay17/1 -> Switch_on18/3
  Delay16/1 -> Switch_on17/3
  Delay15/1 -> Switch_on16/3
  Delay14/1 -> Switch_on15/3
  Delay13/1 -> Switch_on13/3
  Delay12/1 -> Switch_on12/3
  Delay11/1 -> Switch_on11/3
  Delay4/1 -> Switch_on4/3
  Delay10/1 -> Switch_on10/3
  Delay9/1 -> Switch_on9/3
  Delay8/1 -> Switch_on8/3
  Delay3/1 -> Switch_on3/3
  Delay2/1 -> Switch_on2/3
  Delay1/1 -> Switch_on1/3
  Delay33/1 -> Switch_on14/3
